simulink model "Controller_Output"  (R2025b)
settings: Solver=VariableStepAuto  StartTime=0.0  StopTime=inf  RelTol=1e-3
undefined symbols (not defined in the file or in its folder): aileronMax, aileronMin, dirPitch, dirRoll, dirThrottle, dirYaw, elevatorMax, elevatorMin, pitchCh, pitchDB, rollCh, rollDB, throttleCh, throttleDB, uPitchMax, uPitchMin, uRollMax, uRollMin, uThrottleMax, uThrottleMin, uYawMax, uYawMin, yawCh, yawDB
libraries: sl3dlib x1
settings Model: Creator=klakhara  LastModifiedBy=klakhara

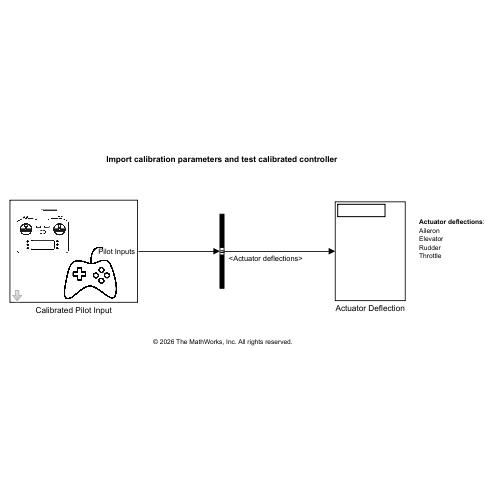
[thumbnail: Simulink's stored preview of the top-level diagram]
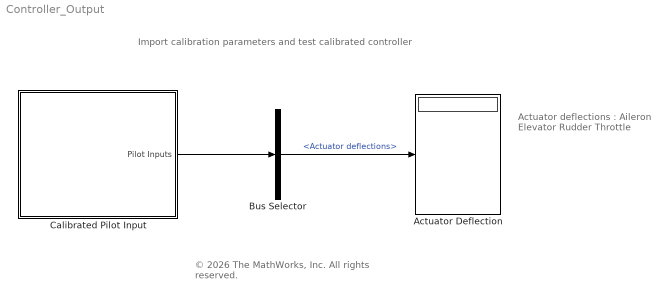
== system Controller_Output ==
  note: Import calibration parameters and test calibrated controller
  note: © 2026 The MathWorks, Inc. All rights reserved.
  note: Actuator deflections :
      | Aileron
      | Elevator
      | Rudder
      | Throttle
  Actuator Deflection : Display
  Bus Selector : BusSelector  OutputSignals=Actuator deflections
  Calibrated Pilot Input : Subsystem  mask{configName=Calibration/Joystick 2.mat, joystickID=Joystick1}
      mask prompts: joystickID "Device ID:"
      mask TypeOptions joystickID: None | Joystick1 | Joystick2 | Joystick3 | Joystick4 | Joystick5 | Joystick6 | Joystick7 | Joystick8 | Joystick9 | Joystick10 | Joystick11 | Joystick12
      mask DialogControl DescGroupVar Prompt: Import calibration parameters to setup the calibreated input device
      mask DialogControl DescTextVar Prompt: Import your calibration configuration file:
      mask DialogControl loadConfig Prompt: Load file
      mask DialogControl ParameterGroupVar Prompt: Identify your Pilot Input Device:
      mask Display: image('Controller_Setup.jpg');
  wires:
  Calibrated Pilot Input/1(Pilot Inputs) -> Bus Selector/1
  Bus Selector/1 -> Actuator Deflection/1  "<Actuator deflections>"

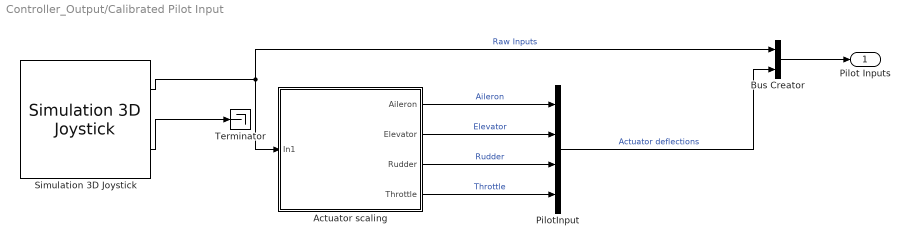
== system Controller_Output/Calibrated Pilot Input ==
  Actuator scaling : Subsystem
  Bus Creator : BusCreator  Inputs=2
  PilotInput : BusCreator  Inputs=4
  Simulation 3D Joystick : sl3dlib/Simulation 3D/Hardware Interface/Simulation 3D Joystick  joyid=1  adjustports=on  forcefeed=off
  Terminator : Terminator
  Pilot Inputs : Outport
  wires:
  Bus Creator/1 -> Pilot Inputs/1
  Simulation 3D Joystick/1 -> Bus Creator/1, Actuator scaling/1(In1)  "Raw Inputs"
  Actuator scaling/2(Elevator) -> PilotInput/2  "Elevator"
  Simulation 3D Joystick/2 -> Terminator/1
  PilotInput/1 -> Bus Creator/2  "Actuator deflections"
  Actuator scaling/3(Rudder) -> PilotInput/3  "Rudder"
  Actuator scaling/4(Throttle) -> PilotInput/4  "Throttle"
  Actuator scaling/1(Aileron) -> PilotInput/1  "Aileron"

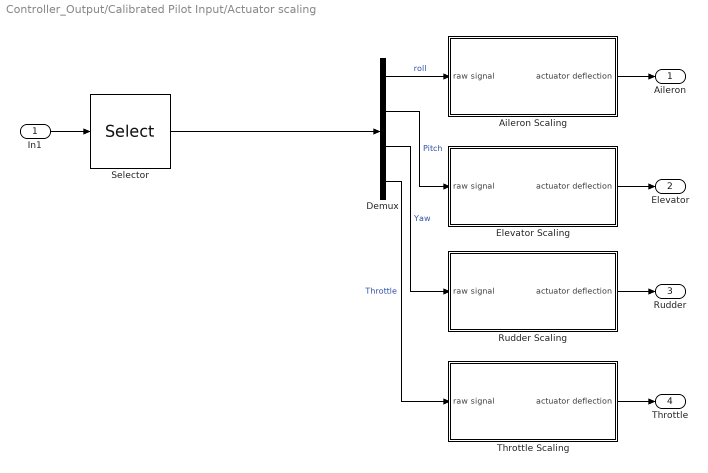
== system Controller_Output/Calibrated Pilot Input/Actuator scaling ==
  In1 : Inport
  Aileron Scaling : Subsystem
  Demux : Demux
  Elevator Scaling : Subsystem
  Rudder Scaling : Subsystem
  Selector : Selector  IndexOptions=Index vector (dialog)  Indices=[rollCh pitchCh yawCh throttleCh]  OutputSizes=1
  Throttle Scaling : Subsystem
  Aileron : Outport
  Elevator : Outport  Port=2
  Rudder : Outport  Port=3
  Throttle : Outport  Port=4
  wires:
  In1/1 -> Selector/1
  Rudder Scaling/1(actuator deflection) -> Rudder/1
  Demux/3 -> Rudder Scaling/1(raw signal)  "Yaw"
  Demux/1 -> Aileron Scaling/1(raw signal)  "roll"
  Selector/1 -> Demux/1
  Elevator Scaling/1(actuator deflection) -> Elevator/1
  Demux/4 -> Throttle Scaling/1(raw signal)  "Throttle"
  Demux/2 -> Elevator Scaling/1(raw signal)  "Pitch"
  Aileron Scaling/1(actuator deflection) -> Aileron/1
  Throttle Scaling/1(actuator deflection) -> Throttle/1

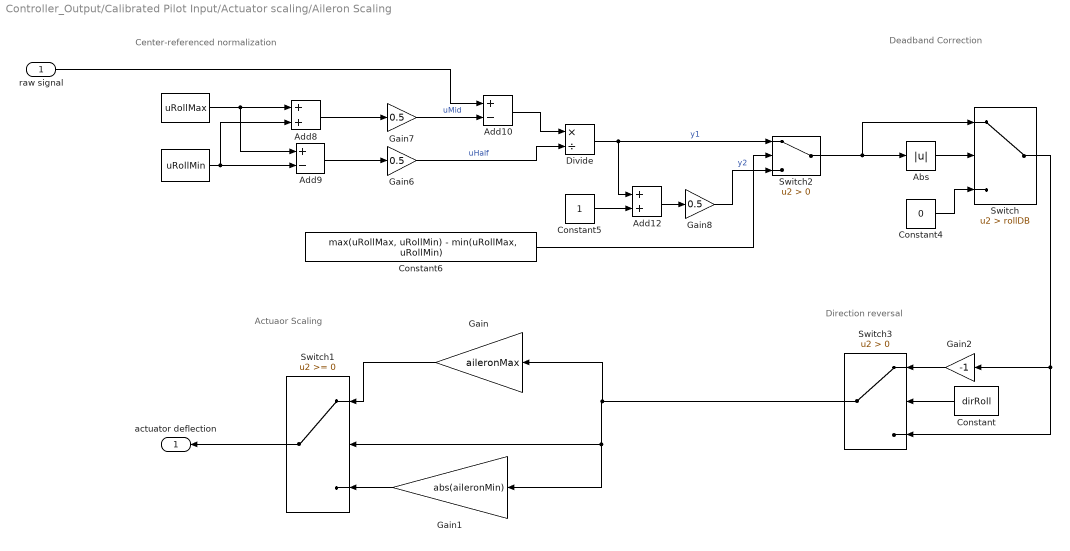
== system Controller_Output/Calibrated Pilot Input/Actuator scaling/Aileron Scaling ==
  note: Direction reversal
  note: Center-referenced normalization
  note: Deadband Correction
  note: Actuaor Scaling
  raw signal : Inport
  " " : Constant  Value=uRollMin
  "   " : Constant  Value=uRollMax
  Abs : Abs  SaturateOnIntegerOverflow=off
  Add10 : Sum  Inputs=+-
  Add12 : Sum
  Add8 : Sum
  Add9 : Sum  Inputs=+-
  Constant : Constant  Value=dirRoll
  Constant4 : Constant  Value=0
  Constant5 : Constant
  Constant6 : Constant  Value=max(uRollMax, uRollMin) - min(uRollMax, uRollMin)
  Divide : Product  Inputs=*/
  Gain : Gain  Gain=aileronMax
  Gain1 : Gain  Gain=abs(aileronMin)
  Gain2 : Gain  Gain=-1
  Gain6 : Gain  Gain=0.5
  Gain7 : Gain  Gain=0.5
  Gain8 : Gain  Gain=0.5
  Switch : Switch  Criteria=u2 > Threshold  Threshold=rollDB  SaturateOnIntegerOverflow=off  InputSameDT=off
  Switch1 : Switch  SaturateOnIntegerOverflow=off  InputSameDT=off
  Switch2 : Switch  Criteria=u2 > Threshold  SaturateOnIntegerOverflow=off  InputSameDT=off
  Switch3 : Switch  Criteria=u2 > Threshold  SaturateOnIntegerOverflow=off  InputSameDT=off
  actuator deflection : Outport
  wires:
  Add9/1 -> Gain6/1
  "   "/1 -> Add9/1, Add8/1
  Add8/1 -> Gain7/1
  " "/1 -> Add8/2, Add9/2
  raw signal/1 -> Add10/1
  Gain7/1 -> Add10/2  "uMid"
  Add10/1 -> Divide/1
  Gain6/1 -> Divide/2  "uHalf"
  Switch1/1 -> actuator deflection/1
  Divide/1 -> Add12/1, Switch2/1  "y1"
  Constant5/1 -> Add12/2
  Add12/1 -> Gain8/1
  Constant6/1 -> Switch2/2
  Gain8/1 -> Switch2/3  "y2"
  Abs/1 -> Switch/2
  Constant4/1 -> Switch/3
  Switch/1 -> Gain2/1, Switch3/3
  Gain/1 -> Switch1/1
  Gain1/1 -> Switch1/3
  Gain2/1 -> Switch3/1
  Switch3/1 -> Gain1/1, Switch1/2, Gain/1
  Constant/1 -> Switch3/2
  Switch2/1 -> Switch/1, Abs/1

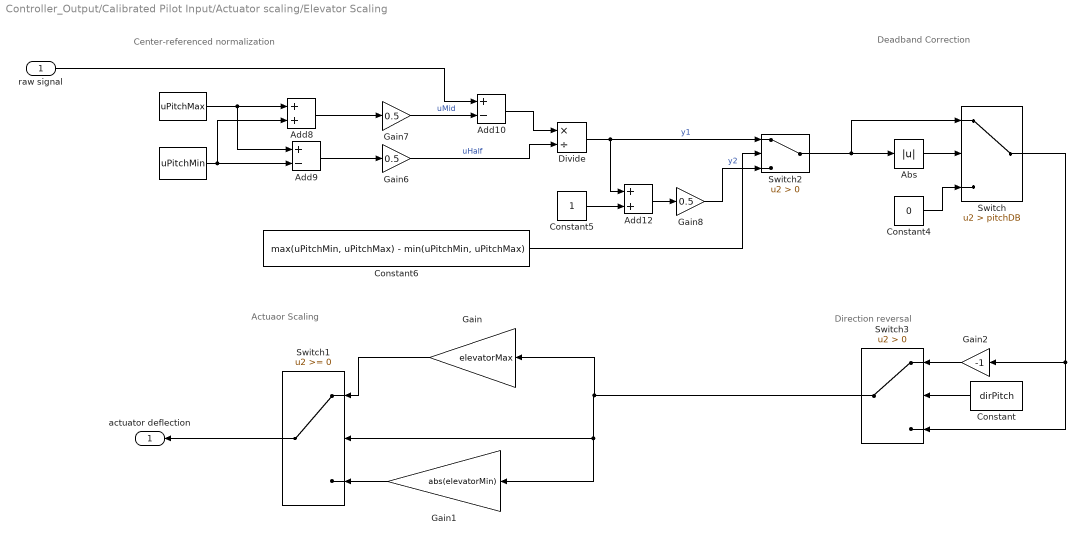
== system Controller_Output/Calibrated Pilot Input/Actuator scaling/Elevator Scaling ==
  note: Direction reversal
  note: Center-referenced normalization
  note: Deadband Correction
  note: Actuaor Scaling
  raw signal : Inport
  " " : Constant  Value=uPitchMin
  "   " : Constant  Value=uPitchMax
  Abs : Abs  SaturateOnIntegerOverflow=off
  Add10 : Sum  Inputs=+-
  Add12 : Sum
  Add8 : Sum
  Add9 : Sum  Inputs=+-
  Constant : Constant  Value=dirPitch
  Constant4 : Constant  Value=0
  Constant5 : Constant
  Constant6 : Constant  Value=max(uPitchMin, uPitchMax) - min(uPitchMin, uPitchMax)
  Divide : Product  Inputs=*/
  Gain : Gain  Gain=elevatorMax
  Gain1 : Gain  Gain=abs(elevatorMin)
  Gain2 : Gain  Gain=-1
  Gain6 : Gain  Gain=0.5
  Gain7 : Gain  Gain=0.5
  Gain8 : Gain  Gain=0.5
  Switch : Switch  Criteria=u2 > Threshold  Threshold=pitchDB  SaturateOnIntegerOverflow=off  InputSameDT=off
  Switch1 : Switch  SaturateOnIntegerOverflow=off  InputSameDT=off
  Switch2 : Switch  Criteria=u2 > Threshold  SaturateOnIntegerOverflow=off  InputSameDT=off
  Switch3 : Switch  Criteria=u2 > Threshold  SaturateOnIntegerOverflow=off  InputSameDT=off
  actuator deflection : Outport
  wires:
  Add9/1 -> Gain6/1
  "   "/1 -> Add9/1, Add8/1
  Add8/1 -> Gain7/1
  " "/1 -> Add8/2, Add9/2
  raw signal/1 -> Add10/1
  Gain7/1 -> Add10/2  "uMid"
  Add10/1 -> Divide/1
  Gain6/1 -> Divide/2  "uHalf"
  Switch1/1 -> actuator deflection/1
  Divide/1 -> Add12/1, Switch2/1  "y1"
  Constant5/1 -> Add12/2
  Add12/1 -> Gain8/1
  Constant6/1 -> Switch2/2
  Gain8/1 -> Switch2/3  "y2"
  Abs/1 -> Switch/2
  Constant4/1 -> Switch/3
  Switch/1 -> Gain2/1, Switch3/3
  Gain/1 -> Switch1/1
  Gain1/1 -> Switch1/3
  Gain2/1 -> Switch3/1
  Switch3/1 -> Gain1/1, Switch1/2, Gain/1
  Constant/1 -> Switch3/2
  Switch2/1 -> Switch/1, Abs/1

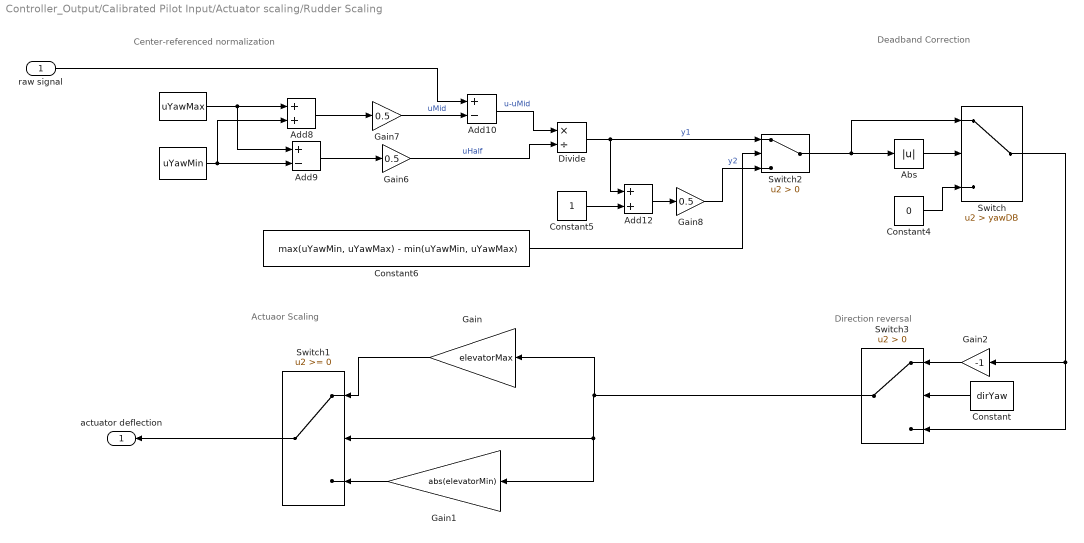
== system Controller_Output/Calibrated Pilot Input/Actuator scaling/Rudder Scaling ==
  note: Direction reversal
  note: Center-referenced normalization
  note: Deadband Correction
  note: Actuaor Scaling
  raw signal : Inport
  " " : Constant  Value=uYawMin
  "   " : Constant  Value=uYawMax
  Abs : Abs  SaturateOnIntegerOverflow=off
  Add10 : Sum  Inputs=+-
  Add12 : Sum
  Add8 : Sum
  Add9 : Sum  Inputs=+-
  Constant : Constant  Value=dirYaw
  Constant4 : Constant  Value=0
  Constant5 : Constant
  Constant6 : Constant  Value=max(uYawMin, uYawMax) - min(uYawMin, uYawMax)
  Divide : Product  Inputs=*/
  Gain : Gain  Gain=elevatorMax
  Gain1 : Gain  Gain=abs(elevatorMin)
  Gain2 : Gain  Gain=-1
  Gain6 : Gain  Gain=0.5
  Gain7 : Gain  Gain=0.5
  Gain8 : Gain  Gain=0.5
  Switch : Switch  Criteria=u2 > Threshold  Threshold=yawDB  SaturateOnIntegerOverflow=off  InputSameDT=off
  Switch1 : Switch  SaturateOnIntegerOverflow=off  InputSameDT=off
  Switch2 : Switch  Criteria=u2 > Threshold  SaturateOnIntegerOverflow=off  InputSameDT=off
  Switch3 : Switch  Criteria=u2 > Threshold  SaturateOnIntegerOverflow=off  InputSameDT=off
  actuator deflection : Outport
  wires:
  Add9/1 -> Gain6/1
  "   "/1 -> Add9/1, Add8/1
  Add8/1 -> Gain7/1
  " "/1 -> Add8/2, Add9/2
  raw signal/1 -> Add10/1
  Gain7/1 -> Add10/2  "uMid"
  Add10/1 -> Divide/1  "u-uMid"
  Gain6/1 -> Divide/2  "uHalf"
  Switch1/1 -> actuator deflection/1
  Divide/1 -> Add12/1, Switch2/1  "y1"
  Constant5/1 -> Add12/2
  Add12/1 -> Gain8/1
  Constant6/1 -> Switch2/2
  Gain8/1 -> Switch2/3  "y2"
  Abs/1 -> Switch/2
  Constant4/1 -> Switch/3
  Switch/1 -> Gain2/1, Switch3/3
  Gain/1 -> Switch1/1
  Gain1/1 -> Switch1/3
  Gain2/1 -> Switch3/1
  Switch3/1 -> Gain1/1, Switch1/2, Gain/1
  Constant/1 -> Switch3/2
  Switch2/1 -> Switch/1, Abs/1

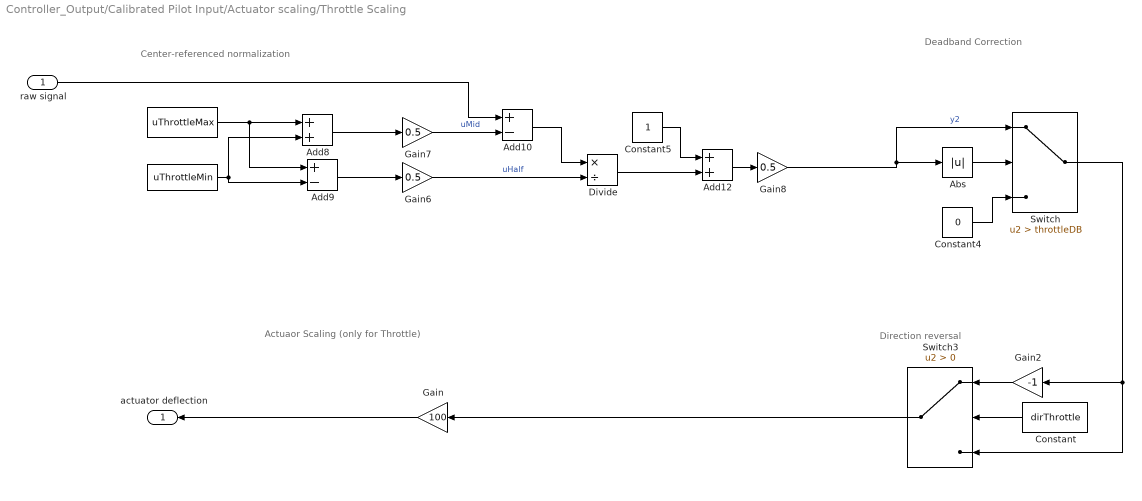
== system Controller_Output/Calibrated Pilot Input/Actuator scaling/Throttle Scaling ==
  note: Direction reversal
  note: Center-referenced normalization
  note: Deadband Correction
  note: Actuaor Scaling (only for Throttle)
  raw signal : Inport
  " " : Constant  Value=uThrottleMin
  "   " : Constant  Value=uThrottleMax
  Abs : Abs  SaturateOnIntegerOverflow=off
  Add10 : Sum  Inputs=+-
  Add12 : Sum
  Add8 : Sum
  Add9 : Sum  Inputs=+-
  Constant : Constant  Value=dirThrottle
  Constant4 : Constant  Value=0
  Constant5 : Constant
  Divide : Product  Inputs=*/
  Gain : Gain  Gain=100
  Gain2 : Gain  Gain=-1
  Gain6 : Gain  Gain=0.5
  Gain7 : Gain  Gain=0.5
  Gain8 : Gain  Gain=0.5
  Switch : Switch  Criteria=u2 > Threshold  Threshold=throttleDB  SaturateOnIntegerOverflow=off  InputSameDT=off
  Switch3 : Switch  Criteria=u2 > Threshold  SaturateOnIntegerOverflow=off  InputSameDT=off
  actuator deflection : Outport
  wires:
  Add9/1 -> Gain6/1
  "   "/1 -> Add9/1, Add8/1
  Add8/1 -> Gain7/1
  " "/1 -> Add9/2, Add8/2
  raw signal/1 -> Add10/1
  Gain7/1 -> Add10/2  "uMid"
  Add10/1 -> Divide/1
  Gain6/1 -> Divide/2  "uHalf"
  Add12/1 -> Gain8/1
  Gain8/1 -> Switch/1, Abs/1  "y2"
  Abs/1 -> Switch/2
  Constant4/1 -> Switch/3
  Switch/1 -> Gain2/1, Switch3/3
  Gain2/1 -> Switch3/1
  Constant/1 -> Switch3/2
  Gain/1 -> actuator deflection/1
  Switch3/1 -> Gain/1
  Constant5/1 -> Add12/1
  Divide/1 -> Add12/2
